simulink library "HANcoder_STM32_Target"  (R2016b)
settings: Solver=ode45  StartTime=0.0  StopTime=10.0  RelTol=1e-3  EnableMultiTasking=on
libraries: simulink x3
(part 4 of 7)

== system HANcoder_STM32_Target/STM32-P405/Digital Outputs ==
  Digital Output : Subsystem  Tag=HANcoder_TARGET_STM32_P405  mask(Digital Output){pinID=Port C pin 12 (LED), config=Push pull, tsamp=-1}
      mask prompts: pinID "Output pin"; config "Configuration"; tsamp "Sample time"
      mask help:
      | Function
      | ========
      | Controls the state of a digital output pin.
      |
      | Parameters
      | ==========
      | Output pin:
      |   Selects the digital output to control
      | Configuration:
      |   Open drain (output float when digital high) or push-pull (output connected
      |   to Vcc when digital high).
      |
      | Inport
      | ==========
      | State of the pin. 0 means logical low and 1 logical high
      mask init:
      | pinIDInfoStr = sfcn_digital_out_mcb(3, pinID, config);
      settings: CopyFcn=sfcn_digital_out_chk();  MoveFcn=drawLogos
      mask Help: web('sfcn_digital_out.html');
      mask TypeOptions pinID: Port A pin 1 | Port A pin 8 | Port B pin 0 | Port B pin 1 | Port B pin 2 | Port B pin 5 | Port B pin 8 | Port B pin 9 | Port B pin 10 | Port B pin 11 | Port B pin 12 | Port B pin 13 | Port B pin 14 | Port B pin 15 | Port C pin 0 | Port C pin 1 | Port C pin 2 | Port C pin 3 | Port C pin 4 | Port C pin 5 | Port C pin 6 | Port C pin 7 | Port C pin 8 | Port C pin 9 | Port C pin 10 | Port C pin 11 | Port C pin 12 (LED) | Port C pin 13 | Port D pin 2
      mask Callback pinID: sfcn_digital_out_chk();
      mask TypeOptions config: Open drain | Push pull
      mask Display: fprintf('Digital Output\n%s', pinIDInfoStr);patch([135 141 141],[8 14 2],[1 0 0]);patch([143 143 149],[14 2 8],[0 0 0.35]);

== system HANcoder_STM32_Target/STM32-P405/Error Handling ==
  Clear errors : Subsystem  Tag=HANcoder_TARGET_STM32_P405  mask(Clear errors){eepromString=Active}
      mask prompts: eepromString "Active or Stored error"
      mask help:
      | [Function]
      | Clears the active(RAM) or stored(EEPROM) errors.
      |
      | [Triggerport]
      | Connect the port to a trigger source to execute the block only when necessary.
      mask init:
      | sfcn_controller_error_clearerrors_mcb(eepromString)
      settings: MoveFcn=drawLogos
      mask Help: web('sfcn_controller_error_clearerrors.html');
      mask TypeOptions eepromString: Active | Stored
      mask Display: fprintf('Clear %s Errors', eepromString);patch([80 86 86],[8 14 2],[1 0 0]);patch([88 88 94],[14 2 8],[0 0 0.35]);
  Delete error : Subsystem  Tag=HANcoder_TARGET_STM32_P405  mask(Delete error){useInPorts=off, errorID=hex2dec('8000'), para=10}
      mask prompts: useInPorts "Use inports"; errorID "Error code"; para "Error parameter"
      mask help:
      | [Function]
      | Delete an error defined by error code and parameter
      | from RAM.
      | Error ID and parameter can be specified in the mask or with inports.
      |
      | [Parameters]
      | Error code
      | Error parameter
      |
      | [Inputs]
      | 1 - Error code [uint16]
      | 2 - Error parameter [uint8]
      |
      | [Triggerport]
      | Connect the port to a trigger source to execute the block only when necessary.
      mask init:
      | sfcn_controller_error_deleteerror_mcb(useInPorts, errorID, para)
      settings: MoveFcn=drawLogos
      mask Help: web('sfcn_controller_error_deleteerror.html');
      mask Display: fprintf('Delete error');patch([80 86 86],[8 14 2],[1 0 0]);patch([88 88 94],[14 2 8],[0 0 0.35]);
  Read active error : Subsystem  Tag=HANcoder_TARGET_STM32_P405  mask(Read active error){tsamp=-1}
      mask prompts: tsamp "Sample time"
      mask help:
      | Function
      | ==========
      | Read an active error from RAM.
      |
      | Inport
      | ==========
      | Input is the number of the error in the error list, which can be 1..64. UINT8
      |
      | Outports
      | ==========
      | 1: UINT8 - total amount of errors.
      | 2: UINT16 - error code.
      | 3: UINT8  - error parameter.
      | 4: UINT8  - occurrence count.
      | 5: UINT32 - last occurrence time since startup [milliseconds].
      |
      | Note that the requested error was set and read only if occurrence count > 0.
      mask init:
      | sfcn_controller_error_readerror_mcb(0)
      settings: MoveFcn=drawLogos
      mask Help: web('sfcn_controller_error_readerror.html');
      mask Display: fprintf('Read active error');patch([80 86 86],[8 14 2],[1 0 0]);patch([88 88 94],[14 2 8],[0 0 0.35]);
  Read stored error : Subsystem  Tag=HANcoder_TARGET_STM32_P405  mask(Read stored error){tsamp=-1}
      mask prompts: tsamp "Sample time"
      mask help:
      | Function
      | ==========
      | Read a stored error from EEPROM.
      |
      | Inport
      | ==========
      | Input is the number of the error in the error list, which can be 1..64. UINT8
      |
      | Outports
      | ==========
      | 1: UINT8 - total amount of errors.
      | 2: UINT16 - error code.
      | 3: UINT8  - error parameter.
      | 4: UINT8  - occurrence count.
      | 5: UINT32 - last occurrence time since startup [milliseconds].
      |
      | Note that the requested error was set and read only if occurrence count > 0.
      mask init:
      | sfcn_controller_error_readerror_mcb(1)
      settings: MoveFcn=drawLogos
      mask Help: web('sfcn_controller_error_readerror.html');
      mask Display: fprintf('Read stored error');patch([80 86 86],[8 14 2],[1 0 0]);patch([88 88 94],[14 2 8],[0 0 0.35]);
  Search active error : Subsystem  Tag=HANcoder_TARGET_STM32_P405  mask(Search active error){tsamp=-1}
      mask prompts: tsamp "Sample time"
      mask help:
      | Function
      | ==========
      | Searches for the erorr with the specified error Code and Param in RAM.
      |
      | Inport
      | ==========
      | 1: UINT16 - Error Code
      | 2: UINT8   - Error Parameter
      |
      | Outports
      | ==========
      | 1: UINT8   - occurrence count.
      | 2: UINT32 - last occurrence time since startup [milliseconds]
      |
      | Note that when occurrence count equals zero, the error is not found.
      mask init:
      | sfcn_controller_error_searcherror_mcb(0)
      settings: MoveFcn=drawLogos
      mask Help: web('sfcn_controller_error_searcherror.html');
      mask Display: fprintf('Search active error');patch([80 86 86],[8 14 2],[1 0 0]);patch([88 88 94],[14 2 8],[0 0 0.35]);
  Search stored error : Subsystem  Tag=HANcoder_TARGET_STM32_P405  mask(Search stored error){tsamp=-1}
      mask prompts: tsamp "Sample time"
      mask help:
      | Function
      | ==========
      | Searches for the erorr with the specified error Code and Param in EEPROM.
      |
      | Inport
      | ==========
      | 1: UINT16 - Error Code
      | 2: UINT8   - Error Parameter
      |
      | Outports
      | ==========
      | 1: UINT8   - occurrence count.
      | 2: UINT32 - last occurrence time since startup [milliseconds]
      |
      | Note that when occurrence count equals zero, the error is not found.
      mask init:
      | sfcn_controller_error_searcherror_mcb(1)
      settings: MoveFcn=drawLogos
      mask Help: web('sfcn_controller_error_searcherror.html');
      mask Display: fprintf('Search stored error');patch([80 86 86],[8 14 2],[1 0 0]);patch([88 88 94],[14 2 8],[0 0 0.35]);
  "Store error " : Subsystem  Tag=HANcoder_TARGET_STM32_P405  mask(Store error){useInPorts=off, errorCode=hex2dec('8000'), parameter=10}
      mask prompts: useInPorts "Use inports"; errorCode "Error code"
      mask help:
      | [Function]
      | Store an error to RAM (and EEPROM if new) of the controller.
      | Error ID and parameter can be specified in the mask or with inports.
      |
      | [Parameters]
      | Error code
      | Error parameter
      |
      | [Inputs]
      | 1 - Error code [uint16]
      | 2 - Error parameter [uint8]
      |
      | [Triggerport]
      | Connect the port to a trigger source to execute the block only when necessary.
      mask init:
      | sfcn_controller_error_storeerror_in_mcb(useInPorts, errorCode, parameter, 1)
      settings: MoveFcn=drawLogos
      mask Help: web('sfcn_controller_error_storeerror.html');
      mask Display: fprintf('Store error');patch([80 86 86],[8 14 2],[1 0 0]);patch([88 88 94],[14 2 8],[0 0 0.35]);
  Total Errors : Subsystem  Tag=HANcoder_TARGET_STM32_P405  mask(Total active or stored errors){eepromString=Active, tsamp=-1}
      mask prompts: eepromString "Active or Stored error"; tsamp "Sample time"
      mask help:
      | [Function]
      | Returns the total amount of active or stored errors
      |
      | [Parameters]
      | Active or Stored error [-]
      | sampleTime: [s]
      |
      | [Outputs]
      | Port 1 :Total number of errors [uint8]
      | Port 2 :Highest occuring severity [uint8]
      mask init:
      | sfcn_controller_error_totalerrors_mcb(eepromString, tsamp);
      settings: MoveFcn=drawLogos
      mask Help: web('sfcn_controller_error_totalerrors.html');
      mask TypeOptions eepromString: Active | Stored
      mask Display: fprintf('Total %s Errors', eepromString);patch([80 86 86],[8 14 2],[1 0 0]);patch([88 88 94],[14 2 8],[0 0 0.35]);

== system HANcoder_STM32_Target/STM32-P405/File Logger ==
  File Logger Close : Subsystem  Tag=HANcoder_TARGET_STM32_P405  mask(File Logger Close){}
      mask help:
      | Function
      | ========
      | With the File Logger module active, the data values of the configured signals
      | are sampled at a fixed time interval and written to the log-file on the SD-card.
      |
      | The log-file needs to be explicitly closed at the end of a logging session for the
      | log-file to actually appear on the SD-card.
      |
      | Ideally, this block is called during software shutdown for example when the ignition
      | signal goes low in automotive applications. An external trigger can also be used such
      | as a button press event or CAN message reception.
      |
      | Triggerport
      | ===========
      | Connect the port to a trigger source to execute the block only when necessary.
      mask init:
      | sfcn_filelogger_close_mcb();
      settings: MoveFcn=drawLogos
      mask Help: web('sfcn_filelogger_close.html')
      mask Display: fprintf('File Logger Close');patch([80 86 86],[8 14 2],[1 0 0]);patch([88 88 94],[14 2 8],[0 0 0.35]);
  File Logger Init : Subsystem  Tag=HANcoder_TARGET_STM32_P405  mask(File Logger Init){filename='mylog.txt', autoincrement=on, firstline='time;signal1;signal2;signal3', interval=100, maxsignals=3, dotseparator=off, autostart=on}
      mask prompts: autoincrement "Add auto-incrementing number to filename"; firstline "First line in log-file"; interval "Logging interval (ms)"; maxsignals "Maximum signals to log"; dotseparator "Use dot-character as decimal separator (comma otherwise)"; autostart "Automatically start logging"
      mask help:
      | Function
      | ==========
      | Initializes the File Logger module.
      |
      | Parameters per channel
      | ======================
      | - Specify filename for the log-file
      | - Select if a 3-digit auto-incrementing number should be added to the log-file
      | - Specify the first line in the log-file
      | - Specify the logging interval in milliseconds
      | - Specify the maximum number of signals to log
      | - Select if a comma or dot should be used a the decimal point in numbers
      | - Select if logging should automatically start after initialization. If not then
      |   a trigger input will appear that can be used to trigger the logging start.
      mask init:
      | sfcn_filelogger_init_mcb(filename, firstline, interval, maxsignals, dotseparator, autoincrement, autostart);
      settings: MoveFcn=drawLogos
      mask Help: web('sfcn_filelogger_init.html')
      mask Display: fprintf('File Logger Init');patch([95 101 101],[8 14 2],[1 0 0]);patch([103 103 109],[14 2 8],[0 0 0.35]);
  File Logger Signal : Subsystem  Tag=HANcoder_TARGET_STM32_P405  mask(File Logger Signal){signalIdx=0, dataType=uint8}
      mask prompts: signalIdx "Signal Index"; dataType "Signal Data Type"
      mask help:
      | Function
      | ==========
      | Configures the signal to be logged by the File Logger module.
      |
      | Parameters per channel
      | ======================
      | - Specify the zero based index of the signal for the File Logger module. In the
      |   File Logger Init block the maximum number of signals was configured
      |   (max_signals). Valid values for this paramter are 0..(max_signals-1).
      | - Select the data type of the signal.
      mask init:
      | sfcn_filelogger_signal_mcb(signalIdx, dataType);
      settings: MoveFcn=drawLogos
      mask Help: web('sfcn_filelogger_signal.html')
      mask TypeOptions dataType: double | single | int8 | uint8 | int16 | uint16 | int32 | uint32
      mask Display: fprintf('File Logger Signal\n(Index %d)', signalIdx);patch([95 101 101],[8 14 2],[1 0 0]);patch([103 103 109],[14 2 8],[0 0 0.35]);

== system HANcoder_STM32_Target/STM32-P405/Memory ==
  EEPROM : Subsystem
      settings: MoveFcn=drawLogos
      mask Display: fprintf('EEPROM');patch([85 91 91],[8 14 2],[1 0 0]);patch([93 93 99],[14 2 8],[0 0 0.35]);

== system HANcoder_STM32_Target/STM32-P405/PWM Outputs ==
  PWM Duty Cycle : Subsystem  Tag=HANcoder_TARGET_STM32_P405  mask(Pulse Width Modulation Set Duty Cycle){pinID=Port A pin 9, tsamp=-1}
      mask prompts: pinID "Output pin"; tsamp "Sample time"
      mask help:
      | Function
      | ========
      | A 'PWM Duty Cycle' block allows the duty cycle of the generated PWM signal to
      | changed.
      | Note that this only works properly if a 'PWM Init' block is also present
      | for initializing the related PWM module.
      |
      | Parameters
      | ==========
      | PWM pin:
      |   Selects the PWM pin for which the duty cycle should be updated.
      |
      | Inport
      | ==========
      | uint16 10-bit unsigned value (0..1023) to represent the duty cycle (0..100%) for
      | each enabled channel.
      mask init:
      | pinIDInfoStr = sfcn_pwmout_setduty_mcb(3, pinID);
      settings: MoveFcn=drawLogos
      mask Help: web('sfcn_pwmout_setduty.html');
      mask TypeOptions pinID: Port A pin 8 | Port A pin 9 | Port A pin 10 | Port A pin 1 | Port C pin 6 | Port C pin 7 | Port C pin 8 | Port C pin 9 | Port B pin 6 | Port B pin 7 | Port B pin 8 | Port B pin 9
      mask Display: fprintf('PWM Set Duty Cycle\n%s', pinIDInfoStr);patch([135 141 141],[8 14 2],[1 0 0]);patch([143 143 149],[14 2 8],[0 0 0.35]);
  PWM Init : Subsystem  Tag=HANcoder_TARGET_STM32_P405  mask(Pulse Width Modulation Initialization){moduleID=TIM1: PA8 & PA9 & PA10 & n/a + N-channels PB13 & PB0 & PB1), frequency=1000, alignment=Edge aligned, enableIRQoutput=off, ch1On=off, ch1Pol=Active high, ch1Inv=off, ch2On=off, ch2Pol=Active high, ch2Inv=off, ch3On=off, ch3Pol=Active high, ch3Inv=off, ch4On=off, ch4Pol=Active high, ch4Inv=off}
      mask prompts: moduleID "PWM module"; frequency "Signal frequency [Hz]"; alignment "Signal alignment"; enableIRQoutput "Enable IRQ output"; ch1On "Generate PWM signal on channel 1"; ch1Pol "Select signal polarity"; ch1Inv "Enable inverted signal on additional output pin"; ch2On "Generate PWM signal on channel 2"; ch2Pol "Select signal polarity"; ch2Inv "Enable inverted signal on additional output pin"; ch3On "Generate PWM signal on channel 3"; ch3Pol "Select signal polarity"; ch3Inv "Enable inverted signal on additional output pin"; ch4On "Generate PWM signal on channel 4"; ch4Pol "Select signal polarity"; ch4Inv "Enable inverted signal on additional output pin"
      mask help:
      | Function
      | ========
      | A 'PWM Init' block configures one of the STM32 timer modules for PWM
      | functionality, allowing a PWM signal to be generated on up to 4 timer
      | channels and their associated output pins.
      |
      | Parameters
      | ==========
      | General - PWM module:
      |   Select the PWM module to use. The name in the combo box contains
      |   information about which pins on the target belong to this timer module.
      |   Also the first pin corresponds with the first channel and so on:
      |   TIMx: Ch1 & Ch2 & Ch3...
      |
      | General - Signal frequency:
      |   Determines the signal frequency in Hz. If you click 'Apply' after entering
      |   the desired frequency it will automatically be adjusted to the closest
      |   supported value.
      |
      | General - Signal Aligment:
      |   Determines the aligment of the signal. It can either be edge aligned or
      |   center aligned.
      |
      | General - Enable IRQ output
      |   Controls whether or not the IRQ output is available.
      |
      | Channel x - Generate PWM signal on channel x:
      |   Enable to configure the channel for PWM functionality so that the PWM signal
      |   is outputted on the channel's associated microcontroller pin.
      |
      | Channel x - Signal polarity:
      |   Selects the polarity of the signal.
      |
      | Channel x - Enable inverted signal on additional output pin:
      |   When enabled, a second PWM signal will be generated on an additional
      |   microcontroller pin where the signal is an exact inversion of the first signal.
      mask init:
      | moduleIDInfoStr = sfcn_pwmout_init_mcb(3, moduleID, frequency, alignment, enableIRQoutput, ch1On, ch2On, ch3On, ch4On, ch1Pol, ch2Pol, ch3Pol, ch4Pol, ch1Inv, ch2Inv, ch3Inv, ch4Inv);
      settings: CopyFcn=sfcn_pwmout_init_chk();  MoveFcn=drawLogos
      mask Help: web('sfcn_pwmout_init.html');
      mask TypeOptions moduleID: TIM1: PA8 & PA9 & PA10 & n/a + N-channels PB13 & PB0 & PB1) | TIM2:n/a & PA1 & n/a & n/a | TIM3: PC6 & PC7 & PC8 & PC9 | TIM4: PB6 & PB7 & PC8 & PB9
      mask Callback moduleID: sfcn_pwmout_init_chk();
      mask TypeOptions alignment: Edge aligned | Center aligned
      mask TypeOptions ch1Pol: Active high | Active low
      mask TypeOptions ch2Pol: Active high | Active low
      mask TypeOptions ch3Pol: Active high | Active low
      mask TypeOptions ch4Pol: Active high | Active low
      mask Display: fprintf('PWM Init\n%s', moduleIDInfoStr);patch([185 191 191],[8 14 2],[1 0 0]);patch([193 193 199],[14 2 8],[0 0 0.35]);

== system HANcoder_STM32_Target/STM32-P405/SPI ==
  SPI master init : Subsystem  Tag=HANcoder_TARGET_STM32_P405  mask(SPI master init){channel=SPI1: UEXT 9 & 7 & 8 (PA5 & PA6 & PA7), speed=5250 kHz, polarity=Idle low, phase=Sample bit on 1st clock edge}
      mask prompts: speed "Communication speed"
      mask help:
      | Function
      | ==========
      | Initialized a SPI master channel.
      |
      | Parameters per channel
      | ======================
      | - Select channel
      | - Select communication speed
      | - Select clock signal polarity
      | - Select clock phase to sample a bit
      mask init:
      | spiChannelInfoStr = sfcn_spi_master_init_mcb(3, channel, speed, polarity, phase);
      settings: CopyFcn=sfcn_spi_master_init_chk();  MoveFcn=drawLogos
      mask Help: web('sfcn_spi_master_init.html')
      mask TypeOptions channel: SPI1: UEXT 9 & 7 & 8 (PA5 & PA6 & PA7) | SPI2: PB13 & PB14 & PB15
      mask Callback channel: sfcn_spi_master_init_chk();
      mask TypeOptions speed: 21000 kHz | 10500 kHz | 5250 kHz | 2625 kHz | 1312.5 kHz | 656.25 kHz | 328.125 kHz | 164.0625 kHz
      mask TypeOptions polarity: Idle low | Idle high
      mask TypeOptions phase: Sample bit on 1st clock edge | Sample bit on 2nd clock edge
      mask Display: fprintf('SPI master init\n%s', spiChannelInfoStr);patch([211 217 217],[8 14 2],[1 0 0]);patch([219 219 225],[14 2 8],[0 0 0.35]);
  SPI master transfer : Subsystem  Tag=HANcoder_TARGET_STM32_P405  mask(SPI master transfer){channel=SPI1: UEXT 9 & 7 & 8 (PA5 & PA6 & PA7), useSS=off, SSpin=Port A pin 1, SSenable=on, SSdisable=on, delayCycles=0, tsamp=-1}
      mask prompts: useSS "Use slave select output"; SSpin "Slave select output pin"; SSenable "Enable slave select before transfer"; SSdisable "Disable slave select after transfer"; delayCycles "Delay cycles between slave select enable and transfer"; tsamp "Sample time"
      mask help:
      | Function
      | ==========
      | Performs a byte transfer via SPI.
      |
      | Parameters per channel
      | ======================
      | - Select channel
      | - Select if a Slave Select output should be controlled
      |   * Select the Slave Select digital output pin
      |   * Select if the Slave Select should be made logic low before the transfer
      |   * Select if the Slave Select should be made logic high after the transfer
      |   * Enter the number of CPU cycles to delay between Slave Select enable and the transfer
      |
      | Inputs
      | ======
      | The byte value to send to the slave.
      |
      | Outputs
      | =======
      | The byte value received from the slave.
      mask init:
      | spiChannelInfoStr = sfcn_spi_master_transfer_mcb(3, channel, useSS, SSpin, SSenable, SSdisable, delayCycles);
      settings: MoveFcn=drawLogos
      mask Help: web('sfcn_spi_master_transfer.html')
      mask TypeOptions channel: SPI1: UEXT 9 & 7 & 8 (PA5 & PA6 & PA7) | SPI2: PB13 & PB14 & PB15
      mask TypeOptions SSpin: Port A pin 1 | Port A pin 8 | Port B pin 0 | Port B pin 1 | Port B pin 2 | Port B pin 5 | Port B pin 8 | Port B pin 9 | Port B pin 10 | Port B pin 11 | Port B pin 12 | Port B pin 13 | Port B pin 14 | Port B pin 15 | Port C pin 0 | Port C pin 1 | Port C pin 2 | Port C pin 3 | Port C pin 4 | Port C pin 5 | Port C pin 6 | Port C pin 7 | Port C pin 8 | Port C pin 9 | Port C pin 10 | Port C pin 11 | Port C pin 12 (LED) | Port C pin 13 | Port D pin 2
      mask Display: fprintf('SPI master transfer\n%s', spiChannelInfoStr);patch([210 216 216],[8 14 2],[1 0 0]);patch([218 218 224],[14 2 8],[0 0 0.35]);

== system HANcoder_STM32_Target/STM32-P405/System Config ==
  Base Sample Time config : Subsystem  Tag=HANcoder_TARGET_STM32_P405  Description=HANcoder Target STM32-P405 blockset version 0.5  mask(Base Sample Time config){baseSampleTime=10, extraStack=100}
      mask prompts: baseSampleTime "Define the base sample time [ms]"; extraStack "Additional task stack (bytes):"
      mask help:
      | Function
      | ==========
      | Sets the Base Sample Time in the model, and automatically sets the sample
      | time in the solver step time menu when the model is simulated or build.
      |
      | Parameters
      | ==========
      | Base Sample Time [milliseconds]
      | Default:    10[ms]
      | Min:        0.1[ms]
      |
      | Note: This is the only block where sample time is set in miliseconds,
      | all other blocks work with sample time in seconds
      |
      | It is possible to reserve extra stack space for the OS task that executes
      | the model on the embedded target (AppCtrlTask).
      mask init:
      | sfcn_base_sample_time_mcb(baseSampleTime*1000, extraStack, 3);
      | HANcoderStruct = get_param(gcb,'UserData');
      | BlocksetVersion = HANcoderStruct.BlocksetVersion;
      settings: MoveFcn=drawLogos
      mask Help: web('sfcn_base_sample_time.html')
      mask Display: fprintf('Blockset version %s\nBase Sample Time:\n %gms',BlocksetVersion,baseSampleTime);patch([91 97 97],[8 14 2],[1 0 0]);patch([99 99 105],[14 2 8],[0 0 0.35]);
  Build settings : Subsystem  Tag=HANcoder_TARGET_STM32_P405  mask(Build Settings){AutoASAP2add=on, AutoFlash=USB}
      mask prompts: AutoASAP2add "Add signals and parameters automatically"; AutoFlash "Automatic flash after build"
      mask help:
      | Function
      | ==========
      | Auto Add:
      | Here you can turn the automatic adding of Signals and Parameters on or off. If the option is on all the parameters and signals which are not defined in the workspace will be added. You will be prompted for the value.
      |
      | Auto Flash:
      | This option will automatically start MicroBoot with the selected interface.
      settings: MoveFcn=drawLogos
      mask Help: web('build_settings.html')
      mask TypeOptions AutoASAP2add: on | off
      mask TypeOptions AutoFlash: off | USB | CAN
      mask DialogControl Control3 Prompt: With this option the undefined parameters and signals will automatically be added to the workspace for use with HANtune. You will be prompted for the parameter values.
      mask DialogControl Control2 Prompt: With this option you can choose to automatically start MicroBoot after the build is complete. MicroBoot will start flashing using the selected interface.
      mask Display: fprintf('Build settings\nAuto Add: %s\nAuto Flash: %s',AutoASAP2add, AutoFlash);patch([114 120 120],[8 14 2],[1 0 0]);patch([122 122 128],[14 2 8],[0 0 0.35]);
  CAN config : Subsystem  Tag=HANcoder_TARGET_STM32_P405  mask(CAN config){txBufSize=64, evBufSize=64, canBus1=on, baudRate1=500, rxMask1=hex2dec('00000000'), rxCode1=hex2dec('00000000'), rxMode1=Receive only 11-bit message identifiers, canBus2=off, baudRate2=500, rxMask2=hex2dec('00000000'), rxCode2=hex2dec('00000000'), rxMode2=Receive only 11-bit message identifiers}
      mask prompts: txBufSize "Transmit buffer size CAN bus (max 512)"; evBufSize "Event buffer size CAN bus"; canBus1 "Use CAN bus 1"; baudRate1 "Baudrate CAN bus 1 (kbit/s)"; rxMask1 "Reception filter Mask CAN bus 1"; rxCode1 "Reception filter Code CAN bus 1"; rxMode1 "Reception filter Mode CAN bus 1"; canBus2 "Use CAN bus 2"; baudRate2 "Baudrate CAN bus 2 (kbit/s)"; rxMask2 "Reception filter Mask CAN bus 2"; rxCode2 "Reception filter Code CAN bus 2"; rxMode2 "Reception filter Mode CAN bus 2"
      mask help:
      | Function
      | ==========
      | Configures the settings for the STM32's CAN busses.
      |
      | Parameters per channel
      | ======================
      | - Activate channel
      | - Select baud rate (default 500[kbit/s])
      | - Select reception acceptance filter Code
      | - Select reception acceptance filter Mask
      | - Select reception acceptance filter Mode
      mask init:
      | sfcn_can_config_mcb(txBufSize, evBufSize, canBus1, baudRate1, rxMask1, rxCode1, rxMode1, canBus2, baudRate2, rxMask2, rxCode2, rxMode2);
      settings: MoveFcn=drawLogos
      mask Help: web('sfcn_can_config.html')
      mask TypeOptions baudRate1: 125 | 250 | 500 | 1000
      mask TypeOptions rxMode1: Receive only 11-bit message identifiers | Receive only 29-bit message identifiers | Received both 11- and 29-bit message identifiers
      mask TypeOptions baudRate2: 125 | 250 | 500 | 1000
      mask TypeOptions rxMode2: Receive only 11-bit message identifiers | Receive only 29-bit message identifiers | Received both 11- and 29-bit message identifiers
      mask Display: fprintf('CAN1 : %x\nCAN2 : %x',canBus1, canBus2);patch([58 64 64],[8 14 2],[1 0 0]);patch([66 66 72],[14 2 8],[0 0 0.35]);
  Custom ID config : Subsystem  Tag=HANcoder_TARGET_STM32_P405  mask(Custom ID config){softID=softwareID, softNUM=1}
      mask prompts: softID "Software ID Name"; softNUM "Software Version Number"
      mask help:
      | Function:
      | =========
      | This block can be used to override the generated software ID as the current software version which is used for identification purposes.
      | It can also be used to add a version number behind the software ID.
      |
      | Details:
      | ========
      | If only a software version number is filled in, a software ID will be generated and the version number will be placed behind it.
      | Atleast one pf the fields has to be filled in.
      |
      | Parameters:
      | ===========
      | Software ID name:
      | Fill in the desired custom ID. Must fit in a UINT8
      | Software Version Number:
      | Fill in the desired version number. Must fit in a UINT8
      mask init:
      | sfcn_custom_version_config_mcb(softID, softNUM)
      settings: MoveFcn=drawLogos
      mask Help: web('sfcn_custom_ID_config.html')
      mask Display: fprintf('Custom software ID:\n "%s"\n Software version:\n "%s"', char(softID), char(softNUM));patch([112 118 118],[8 14 2],[1 0 0]);patch([120 120 126],[14 2 8],[0 0 0.35]);
  XCP on CAN config : Subsystem  Tag=HANcoder_TARGET_STM32_P405  mask(XCP on CAN config){canBus=CAN 1, croID=hex2dec('665'), dtoID=hex2dec('666')}
      mask prompts: canBus "CAN channel"; croID "CRO identifier"; dtoID "DTO identifier"
      mask help:
      | Function
      | ==========
      | Implements XCP communication into your application using the CAN network.
      |
      | Parameter
      | ==========
      | Specify the CAN channel to be used for XCP.
      | Specify the CAN CRO message identifier for XCP (master->slave).
      | Specify the CAN DTO message identifier for XCP (slave->master).
      |
      | Notes
      | ==========
      | Baudrates can be modified in the CAN config block.
      mask init:
      | sfcn_can_xcp_config_mcb(canBus, croID, dtoID)
      settings: MoveFcn=drawLogos
      mask Help: web('sfcn_can_xcp_config.html')
      mask TypeOptions canBus: CAN 1 | CAN 2
      mask Display: fprintf('XCP over CAN: %x',canBus);patch([69 75 75],[8 14 2],[1 0 0]);patch([77 77 83],[14 2 8],[0 0 0.35]);
  XCP on USB config : Subsystem  Tag=HANcoder_TARGET_STM32_P405  mask(XCP on USB config){}
      mask help:
      | Function
      | ==========
      | Implements XCP communication into your application using the USB Virtual COM-port.
      mask init:
      | sfcn_usb_xcp_config_mcb()
      settings: MoveFcn=drawLogos
      mask Help: web('sfcn_usb_xcp_config.html')
      mask Display: fprintf('XCP over USB');patch([69 75 75],[8 14 2],[1 0 0]);patch([77 77 83],[14 2 8],[0 0 0.35]);

== system HANcoder_STM32_Target/STM32-P405/System Management ==
  Enter Critical Section : Subsystem  Tag=HANcoder_TARGET_STM32_P405  mask(Enter a critical section){tsamp=-1}
      mask prompts: tsamp "Sample time"
      mask help:
      | Function
      | ==========
      | Enters a critical section that can not be interrupted. This block must
      | always be used in a pair together with "Exit Critical Section". Click the
      | Help-button for a detailed example on how to use this block.
      mask init:
      | sfcn_critical_enter_mcb();
      settings: MoveFcn=drawLogos
      mask Help: web('sfcn_critical_section.html');
      mask Display: fprintf('Enter Critical Section');patch([95 101 101],[8 14 2],[1 0 0]);patch([103 103 109],[14 2 8],[0 0 0.35]);
  Exit Critical Section : Subsystem  Tag=HANcoder_TARGET_STM32_P405  mask(Exit a critical section){tsamp=-1}
      mask prompts: tsamp "Sample time"
      mask help:
      | Function
      | ==========
      | Exits a critical section. This block must always be used in a pair together
      | with "Enter Critical Section". Click the Help-button for a detailed example
      | on how to use this block.
      mask init:
      | sfcn_critical_exit_mcb();
      settings: MoveFcn=drawLogos
      mask Help: web('sfcn_critical_section.html');
      mask Display: fprintf('Exit Critical Section');patch([95 101 101],[8 14 2],[1 0 0]);patch([103 103 109],[14 2 8],[0 0 0.35]);
  Get CPU load : Subsystem  Tag=HANcoder_TARGET_STM32_P405  mask(Get CPU load){mode=Current CPU load, tsamp=-1}
      mask prompts: tsamp "Sample time"
      mask help:
      | Function
      | ==========
      | Get the CPU load of the system.
      |
      | Parameters
      | ==========
      | Mode specifies if the current CPU load should be read or the maximum CPU
      | load since reset.
      |
      | Outport
      | ==========
      | CPU load as a percentage.
      mask init:
      | if mode==1
      |   modeStr = 'current';
      | else
      |   modeStr = 'maximum';
      | end
      | sfcn_controller_cpu_getload_mcb(mode);
      settings: MoveFcn=drawLogos
      mask Help: web('sfcn_controller_cpu_getload.html');
      mask TypeOptions mode: Current CPU load | Maximum CPU load
      mask Display: fprintf('Get %s\nCPU load', modeStr);patch([95 101 101],[8 14 2],[1 0 0]);patch([103 103 109],[14 2 8],[0 0 0.35]);
  Get free Heap : Subsystem  Tag=HANcoder_TARGET_STM32_P405  mask(Get free Heap){tsamp=-1}
      mask prompts: tsamp "Sample time"
      mask help:
      | Function
      | ==========
      | Obtains the number of bytes that are still available on the heap.
      |
      | Outport
      | ==========
      | Number of bytes that are still available on the heap.
      mask init:
      | sfcn_controller_getheap_mcb();
      settings: MoveFcn=drawLogos
      mask Help: web('sfcn_controller_getheap.html');
      mask Display: fprintf('Get free Heap');patch([95 101 101],[8 14 2],[1 0 0]);patch([103 103 109],[14 2 8],[0 0 0.35]);
  Get free Stack : Subsystem  Tag=HANcoder_TARGET_STM32_P405  mask(Get free Stacl){taskIdx=Application Control Task, tsamp=-1}
      mask prompts: taskIdx "Task name"; tsamp "Sample time"
      mask help:
      | Function
      | ========
      | Obtains the number of bytes that are still available on the stack of a particular task.
      |
      | Parameter
      | =========
      | Name of the task for which the free stack space should be read.
      |
      | Outport
      | =======
      | Number of bytes that are still available on the task's stack.
      mask init:
      | sfcn_controller_getstack_mcb(taskIdx);
      settings: MoveFcn=drawLogos
      mask Help: web('sfcn_controller_getstack.html');
      mask TypeOptions taskIdx: Idle Task | Timer Task | Can Event Task | Can Transmit Task | Application Control Task | Measurement and Calibration Network Task
      mask Display: fprintf('Get free Stack');patch([95 101 101],[8 14 2],[1 0 0]);patch([103 103 109],[14 2 8],[0 0 0.35]);
  Reset ECU : Subsystem  Tag=HANcoder_TARGET_STM32_P405  mask(Reset ECU){}
      mask help:
      | Function
      | ==========
      | Triggering this block causes the ECU to reset.
      mask init:
      | sfcn_controller_reset_mcb()
      settings: MoveFcn=drawLogos
      mask Help: web('sfcn_controller_reset.html');
      mask Display: fprintf('Reset ECU');patch([60 66 66],[8 14 2],[1 0 0]);patch([68 68 74],[14 2 8],[0 0 0.35]);

== system HANcoder_STM32_Target/STM32-P405/Timer Inputs ==
  Quadrature Encoder Get : Subsystem  Tag=HANcoder_TARGET_STM32_P405  mask(Quadrature Encoder Inputs){moduleID=TIM3: PORTC PIN6 & PORTC PIN7 - 5V Tolerant, config=Floating, counterReset=off, tsamp=-1}
      mask prompts: moduleID "Quad encoder module"; config "Configuration"; counterReset "Show counter reset input"; tsamp "Sample time"
      mask help:
      | Function
      | ========
      | Reads the counter of the quadrature encoder module.
      |
      | Parameters
      | ==========
      | Quadrature encoder module:
      |   Selects the quadrature encoder module. The channel A and B signals of the
      |   encoder should be connected to the 2 input pins that belong to the module.
      |
      | Configuration:
      |   Determines if the input is floating or is connected to an internal
      |   pull-up or pull-down resistor.
      |
      | Show counter reset input:
      |   Configures if the input port for the counter reset should be shown.
      |
      |
      | Outport
      | ==========
      | 32-bit signed counter. The counter starts at zero and counts up or down
      | depending on the direction of the motor.
      mask init:
      | moduleIDInfoStr = sfcn_quad_encoder_get_mcb(3,moduleID, counterReset, config);
      settings: CopyFcn=sfcn_quad_encoder_get_chk();  MoveFcn=drawLogos
      mask Help: web('sfcn_quad_encoder_get.html');
      mask TypeOptions moduleID: TIM1: PORTA PIN8 & PORTA PIN9 - 5V Tolerant | TIM3: PORTC PIN6 & PORTC PIN7 - 5V Tolerant | TIM4: PORTB PIN6 & PORTB PIN7 - 5V Tolerant
      mask Callback moduleID: sfcn_quad_encoder_get_chk();
      mask TypeOptions config: Floating | Pullup | Pulldown
      mask Display: fprintf('Quad Encoder Get\n%s', moduleIDInfoStr);patch([135 141 141],[8 14 2],[1 0 0]);patch([143 143 149],[14 2 8],[0 0 0.35]);
  Timer Input Get : Subsystem  Tag=HANcoder_TARGET_STM32_P405  mask(Timer Input Get){pin=TIM1: Con. PA8 (PORTA PIN8) - 5V Tolerant, zeroHzTimeoutMs=2000, tsamp=-1}
      mask prompts: pin "Timer input pin"; zeroHzTimeoutMs "0 Hz detection time (ms)"; tsamp "Sample time"
      mask help:
      | Function
      | ========
      | Reads the information from a timer input pin.
      |
      | Parameters
      | ==========
      | Timer input pin:
      |   Selects the timer input pin.
      |
      | Zero Hz detection time:
      |   Determines after how many milliseconds since the last edge the 0 Hz
      |   detected output flag should go high.
      |
      | Outport
      | ==========
      | Frequency
      |   The last measured frequency on the pin in Hz.
      |
      | Duty cycle
      |   The last measured duty cycle on the pin as a % with a scaling factor of 100 for
      |   improved resolution. So 5000 = 50% for example.
      |
      | Edge count
      |   The number of edges that were detected on the input pin since startup.
      |
      | Edge timestamp
      |   A 32-bit timestamp value of the last edge. The timestamp is derived from an
      |   internal 32-bit free running counter that runs at 21 Mhz.
      |
      | 0 Hz detected
      |   A boolean flag that will go high if no edges were detected for the time specified
      |   as the zero Hz detection time. Upon the next edge the flag will go low again.
      mask init:
      | timeinPinIdInfoStr = sfcn_timein_get_mcb(3, pin, zeroHzTimeoutMs);
      settings: CopyFcn=sfcn_timein_get_chk();  MoveFcn=drawLogos
      mask Help: web('sfcn_timein_get.html');
      mask TypeOptions pin: TIM1: Con. PA8 (PORTA PIN8) - 5V Tolerant | TIM1: Con. UEXT-3 (PORTA PIN9) - 5V Tolerant | TIM1: Con. UEXT-4 (PORTA PIN10) - 5V Tolerant | TIM2: Con. PA1 (PORTA PIN1) - 5V Tolerant | TIM3: Con. PC6 (PORTC PIN6) - 5V Tolerant | TIM3: Con. PC7 (PORTC PIN7) - 5V Tolerant | TIM3: Con. PC8 (PORTC PIN8) - 5V Tolerant | TIM3: Con. PC9 (PORTC PIN9) - 5V Tolerant | TIM4: Con. UEXT-5 (PORTB PIN6) - 5V Tolerant | TIM4: Con. UEXT-6 (PORTB PIN7) - 5V Tolerant | TIM4: Con. PB8 (PORTB PIN8) - 5V Tolerant | TIM4: Con. PB9 (PORTB PIN9) - 5V Tolerant
      mask Callback pin: sfcn_timein_get_chk();
      mask Display:
      | fprintf('Timer Input Get\n%s', timeinPinIdInfoStr);
      | port_label('output', 1, 'Frequency');
      | port_label('output', 2, 'Duty cycle');
      | port_label('output', 3, 'Edge count');
      | port_label('output', 4, 'Edge state');
      | port_label('output', 5, 'Edge timestamp');
      | port_label('output', 6, 'Counter timestamp');
      | port_label('output', 7, '0 Hz detected');patch([250 256 256],[8 14 2],[1 0 0]);patch([258 258 264],[14 2 8],[0 0 0.35]);
  Timer Input IRQ : Subsystem  Tag=HANcoder_TARGET_STM32_P405  mask(Timer Input IRQ){pin=TIM1: Con. PA8 (PORTA PIN8) - 5V Tolerant}
      mask prompts: pin "Timer input pin"
      mask help:
      | Function
      | ========
      | Enables a function call subsystem to be connected that is executed on interrupt level
      | each time an edge change on the input pin was detected.
      |
      | Parameters
      | ==========
      | Timer input pin:
      |   Selects the timer input pin.
      |
      | Outport
      | =======
      | IRQ
      |   Allows connection of a function call subsystem.
      mask init:
      | timeinPinIdInfoStr = sfcn_timein_irq_mcb(3, pin);
      settings: CopyFcn=sfcn_timein_irq_chk();  MoveFcn=drawLogos
      mask Help: web('sfcn_timein_irq.html');
      mask TypeOptions pin: TIM1: Con. PA8 (PORTA PIN8) - 5V Tolerant | TIM1: Con. UEXT-3 (PORTA PIN9) - 5V Tolerant | TIM1: Con. UEXT-4 (PORTA PIN10) - 5V Tolerant | TIM2: Con. PA1 (PORTA PIN1) - 5V Tolerant | TIM3: Con. PC6 (PORTC PIN6) - 5V Tolerant | TIM3: Con. PC7 (PORTC PIN7) - 5V Tolerant | TIM3: Con. PC8 (PORTC PIN8) - 5V Tolerant | TIM3: Con. PC9 (PORTC PIN9) - 5V Tolerant | TIM4: Con. UEXT-5 (PORTB PIN6) - 5V Tolerant | TIM4: Con. UEXT-6 (PORTB PIN7) - 5V Tolerant | TIM4: Con. PB8 (PORTB PIN8) - 5V Tolerant | TIM4: Con. PB9 (PORTB PIN9) - 5V Tolerant
      mask Callback pin: sfcn_timein_irq_chk();
      mask Display: fprintf('Timer Input IRQ\n%s', timeinPinIdInfoStr);patch([250 256 256],[8 14 2],[1 0 0]);patch([258 258 264],[14 2 8],[0 0 0.35]);

== system HANcoder_STM32_Target/STM32-P405/Timer Outputs ==
  Compare Event IRQ : Subsystem  Tag=HANcoder_TARGET_STM32_P405  mask(Compare Event IRQ){pin=TIM1: Con. PA8 (PORTA PIN8) - 5V Tolerant}
      mask prompts: pin "Timer output pin"
      mask help:
      | Function
      | ========
      | Enables a function call subsystem to be connected that is executed on interrupt
      | level each time an output compare event was triggered.
      |
      | Parameters
      | ==========
      | Timer Output Pin:
      |   Selects the timer channel.
      |
      | Outport
      | =======
      | IRQ
      |   Allows connection of a function call subsystem.
      mask init:
      | timeoutPinIdInfoStr = sfcn_timeout_event_irq_mcb(3, pin);
      settings: CopyFcn=sfcn_timeout_event_irq_chk();  MoveFcn=drawLogos
      mask Help: web('sfcn_timeout_event_irq.html');
      mask TypeOptions pin: TIM1: Con. PA8 (PORTA PIN8) - 5V Tolerant | TIM1: Con. UEXT-3 (PORTA PIN9) - 5V Tolerant | TIM1: Con. UEXT-4 (PORTA PIN10) - 5V Tolerant | TIM2: Con. PA1 (PORTA PIN1) - 5V Tolerant | TIM3: Con. PC6 (PORTC PIN6) - 5V Tolerant | TIM3: Con. PC7 (PORTC PIN7) - 5V Tolerant | TIM3: Con. PC8 (PORTC PIN8) - 5V Tolerant | TIM3: Con. PC9 (PORTC PIN9) - 5V Tolerant | TIM4: Con. UEXT-5 (PORTB PIN6) - 5V Tolerant | TIM4: Con. UEXT-6 (PORTB PIN7) - 5V Tolerant | TIM4: Con. PB8 (PORTB PIN8) - 5V Tolerant | TIM4: Con. PB9 (PORTB PIN9) - 5V Tolerant
      mask Callback pin: sfcn_timeout_event_irq_chk();
      mask Display: fprintf('Compare Event IRQ\n%s', timeoutPinIdInfoStr);patch([135 141 141],[8 14 2],[1 0 0]);patch([143 143 149],[14 2 8],[0 0 0.35]);
  Get Free Running Counter : Subsystem  Tag=HANcoder_TARGET_STM32_P405  mask(Get Free Running Counter){moduleID=TIM1, tsamp=-1}
      mask prompts: moduleID "Timer module"; tsamp "Sample time"
      mask help:
      | Function
      | ========
      | Reads the timer module's internal 16-bit free running counter value.
      |
      | Parameters
      | ==========
      | Timer Module:
      |   Selects the timer module.
      |
      | Outport
      | =======
      | 16-bit free running counter value.
      mask init:
      | moduleIDInfoStr = sfcn_timeout_getrunningcounter_mcb(3, moduleID);
      settings: MoveFcn=drawLogos
      mask Help: web('sfcn_timeout_getrunningcounter.html');
      mask TypeOptions moduleID: TIM1 | TIM2 | TIM3 | TIM4
      mask Display: fprintf('Get Free Running Counter\n%s', moduleIDInfoStr);patch([135 141 141],[8 14 2],[1 0 0]);patch([143 143 149],[14 2 8],[0 0 0.35]);
  Get Last Event Counter : Subsystem  Tag=HANcoder_TARGET_STM32_P405  mask(Get Last Event Counter){pin=TIM1: Con. PA8 (PORTA PIN8) - 5V Tolerant, tsamp=-1}
      mask prompts: pin "Timer output pin"; tsamp "Sample time"
      mask help:
      | Function
      | ========
      | Reads the timer channel's timestamp of the 16-bit free running counter
      | value at which the last output compare event occurred.
      |
      | Parameters
      | ==========
      | Timer Output Pin:
      |   Selects the timer channel.
      |
      | Outport
      | =======
      | 16-bit free running counter timestamp of the last output compare event.
      mask init:
      | timeoutPinIdInfoStr = sfcn_timeout_getlasteventcounter_mcb(3, pin);
      settings: MoveFcn=drawLogos
      mask Help: web('sfcn_timeout_getlasteventcounter.html');
      mask TypeOptions pin: TIM1: Con. PA8 (PORTA PIN8) - 5V Tolerant | TIM1: Con. UEXT-3 (PORTA PIN9) - 5V Tolerant | TIM1: Con. UEXT-4 (PORTA PIN10) - 5V Tolerant | TIM2: Con. PA1 (PORTA PIN1) - 5V Tolerant | TIM3: Con. PC6 (PORTC PIN6) - 5V Tolerant | TIM3: Con. PC7 (PORTC PIN7) - 5V Tolerant | TIM3: Con. PC8 (PORTC PIN8) - 5V Tolerant | TIM3: Con. PC9 (PORTC PIN9) - 5V Tolerant | TIM4: Con. UEXT-5 (PORTB PIN6) - 5V Tolerant | TIM4: Con. UEXT-6 (PORTB PIN7) - 5V Tolerant | TIM4: Con. PB8 (PORTB PIN8) - 5V Tolerant | TIM4: Con. PB9 (PORTB PIN9) - 5V Tolerant
      mask Display: fprintf('Get Last Event Counter\n%s', timeoutPinIdInfoStr);patch([135 141 141],[8 14 2],[1 0 0]);patch([143 143 149],[14 2 8],[0 0 0.35]);
  Output Compare Init : Subsystem  Tag=HANcoder_TARGET_STM32_P405  mask(Output Compare Init){moduleID=TIM1: PA8 & PA9 & PA10 & n/a, frequency=2000000, enableIRQoutput=off}
      mask prompts: moduleID "Timer module"; frequency "Frequency (free running counter) [Hz]"; enableIRQoutput "Enable IRQ output"
      mask help:
      | Function
      | ========
      | Initializes the timer module to allow output compare functionality on the
      | module's channels.
      |
      | Parameters
      | ==========
      | Timer Module:
      |   Selects the timer module.
      |
      | Frequency:
      |   Frequency at which the 16-bit free running counter counts.
      |
      | Enable IRQ output
      |   Controls whether or not the IRQ output is available.
      |
      | Outport
      | =======
      | IRQ
      |   Allows connection of a function call subsystem for the free running
      |   counter overflow event.
      mask init:
      | moduleIDInfoStr = sfcn_timeout_init_mcb(3, moduleID, frequency, enableIRQoutput);
      settings: CopyFcn=sfcn_timeout_init_chk();  MoveFcn=drawLogos
      mask Help: web('sfcn_timeout_init.html');
      mask TypeOptions moduleID: TIM1: PA8 & PA9 & PA10 & n/a | TIM2: n/a & PA1 & n/a & n/a | TIM3: PC6 & PC7 & PC8 & PC9 | TIM4: PB6 & PB7 & PC8 & PB9
      mask Callback moduleID: sfcn_timeout_init_chk();
      mask Display: fprintf('Output Compare Init\n%s', moduleIDInfoStr);patch([135 141 141],[8 14 2],[1 0 0]);patch([143 143 149],[14 2 8],[0 0 0.35]);
  Reset Free Running Counter : Subsystem  Tag=HANcoder_TARGET_STM32_P405  mask(Reset Free Running Counter){moduleID=TIM1}
      mask prompts: moduleID "Timer module"
      mask help:
      | Function
      | ========
      | Resets the value of the timer module's 16-bit free running counter back to
      | 0.
      |
      | Triggerport
      | ===========
      | Connect the port to a trigger source to execute the block only when necessary.
      mask init:
      | moduleIDInfoStr = sfcn_timeout_resetcounter_mcb(3, moduleID);
      settings: MoveFcn=drawLogos
      mask Help: web('sfcn_timeout_resetcounter.html');
      mask TypeOptions moduleID: TIM1 | TIM2 | TIM3 | TIM4
      mask Display: fprintf('Reset Free Running Counter\n%s', moduleIDInfoStr);patch([132 138 138],[8 14 2],[1 0 0]);patch([140 140 146],[14 2 8],[0 0 0.35]);
  Schedule Compare Event : Subsystem  Tag=HANcoder_TARGET_STM32_P405  mask(Schedule Compare Event){pin=TIM1: Con. PA8 (PORTA PIN8) - 5V Tolerant, tsamp=-1}
      mask prompts: pin "Timer output pin"; tsamp "Sample time"
      mask help:
      | Function
      | ========
      | Schedules the next output compare event. The first input determines the
      | value of the timer module's 16-bit free running counter when the event
      | should trigger. The second input determines the action that should
      | be taken on the timer channel's pin.
      |
      | Parameters
      | ==========
      | Timer output pin:
      |   Selects the timer channel's pin.
      |
      | Inport
      | ======
      | Counter
      |   Value of the timer module's 16-bit free running counter at which the
      |   event should trigger.
      |
      | Action
      |   Action to take on the channel's pin when the event triggers:
      |   0: set output pin to logic low.
      |   1: set output pin to logic high.
      |   2: invert logic state of the outpin pin.
      |   3: do nothing to the output pin.
      mask init:
      | timeoutPinIdInfoStr = sfcn_timeout_scheduleevent_mcb(3, pin);
      settings: MoveFcn=drawLogos
      mask Help: web('sfcn_timeout_scheduleevent.html');
      mask TypeOptions pin: TIM1: Con. PA8 (PORTA PIN8) - 5V Tolerant | TIM1: Con. UEXT-3 (PORTA PIN9) - 5V Tolerant | TIM1: Con. UEXT-4 (PORTA PIN10) - 5V Tolerant | TIM2: Con. PA1 (PORTA PIN1) - 5V Tolerant | TIM3: Con. PC6 (PORTC PIN6) - 5V Tolerant | TIM3: Con. PC7 (PORTC PIN7) - 5V Tolerant | TIM3: Con. PC8 (PORTC PIN8) - 5V Tolerant | TIM3: Con. PC9 (PORTC PIN9) - 5V Tolerant | TIM4: Con. UEXT-5 (PORTB PIN6) - 5V Tolerant | TIM4: Con. UEXT-6 (PORTB PIN7) - 5V Tolerant | TIM4: Con. PB8 (PORTB PIN8) - 5V Tolerant | TIM4: Con. PB9 (PORTB PIN9) - 5V Tolerant
      mask Display: fprintf('Schedule Compare Event\n%s', timeoutPinIdInfoStr);patch([135 141 141],[8 14 2],[1 0 0]);patch([143 143 149],[14 2 8],[0 0 0.35]);

== system HANcoder_STM32_Target/STM32-P405/UART ==
  UART init : Subsystem  Tag=HANcoder_TARGET_STM32_P405  mask(UART init){channel=UART1: Con. UEXT-3 & Con. UEXT-4 (PA9 & PA10), baudrate=19200, databits=8, parity=none, stopbits=1, txbufsize=32, rxbufsize=32, useStatusOut=off}
      mask prompts: baudrate "Baudrate (bit/s)"; txbufsize "Transmit buffer size"; rxbufsize "Receive buffer size"; useStatusOut "Use status output"
      mask help:
      | Function
      | ==========
      | Initialized a UART channel.
      |
      | Parameters per channel
      | ======================
      | - Select channel
      | - Select baudrate
      | - Select number of databits
      | - Select parity
      | - Select number of stopbits
      | - Configure the size of the transmit buffer
      | - Configure the size of the reception buffer
      | - Enable/disable the status output port
      mask init:
      | uartChannelInfoStr = sfcn_uart_init_mcb(3, channel, baudrate, databits, parity, stopbits, txbufsize, rxbufsize, useStatusOut);
      settings: CopyFcn=sfcn_uart_init_chk();  MoveFcn=drawLogos
      mask Help: web('sfcn_uart_init.html')
      mask TypeOptions channel: UART1: Con. UEXT-3 & Con. UEXT-4 (PA9 & PA10) | UART2: SUB D9 (PA2 & PA3)
      mask Callback channel: sfcn_uart_init_chk();
      mask TypeOptions baudrate: 300 | 600 | 1200 | 2400 | 4800 | 9600 | 19200 | 38400 | 57600 | 115200
      mask TypeOptions databits: 8 | 9
      mask TypeOptions parity: none | even | odd
      mask TypeOptions stopbits: 1 | 2
      mask Display: fprintf('UART init\n%s', uartChannelInfoStr);patch([236 242 242],[8 14 2],[1 0 0]);patch([244 244 250],[14 2 8],[0 0 0.35]);
  UART receive : Subsystem  Tag=HANcoder_TARGET_STM32_P405  mask(UART receive){channel=UART1: Con. UEXT-3 & Con. UEXT-4 (PA9 & PA10), useStatusOut=off, tsamp=-1}
      mask prompts: useStatusOut "Use status outport"; tsamp "Sample time"
      mask help:
      | Function
      | ==========
      | Reads a byte from the UART reception buffer.
      |
      | Parameters per channel
      | ======================
      | - Select channel
      | - Select if the status output should be enabled.
      |
      | Outputs
      | =======
      | - The value of the receive byte.
      | - When the status output is 0, the reception buffer was empty.
      mask init:
      | uartChannelInfoStr = sfcn_uart_receive_mcb(3, channel, useStatusOut);
      settings: MoveFcn=drawLogos
      mask Help: web('sfcn_uart_receive.html')
      mask TypeOptions channel: UART1: Con. UEXT-3 & Con. UEXT-4 (PA9 & PA10) | UART2: SUB D9 (PA2 & PA3)
      mask Display: fprintf('UART receive\n%s', uartChannelInfoStr);patch([240 246 246],[8 14 2],[1 0 0]);patch([248 248 254],[14 2 8],[0 0 0.35]);
  UART receive buffer status : Subsystem  Tag=HANcoder_TARGET_STM32_P405  mask(UART receive buffer status){channel=UART1: Con. UEXT-3 & Con. UEXT-4 (PA9 & PA10), tsamp=-1}
      mask prompts: tsamp "Sample time"
      mask help:
      | Function
      | ==========
      | Obtains the number of received bytes that are currently stored in the
      | reception buffer.
      |
      | Parameters per channel
      | ======================
      | - Select channel
      |
      | Outputs
      | ======
      | - The number of bytes currently stored in the reception buffer.
      mask init:
      | uartChannelInfoStr = sfcn_uart_receive_size_mcb(3, channel);
      settings: MoveFcn=drawLogos
      mask Help: web('sfcn_uart_receive_size.html')
      mask TypeOptions channel: UART1: Con. UEXT-3 & Con. UEXT-4 (PA9 & PA10) | UART2: SUB D9 (PA2 & PA3)
      mask Display: fprintf('UART receive buffer status\n%s', uartChannelInfoStr);patch([245 251 251],[8 14 2],[1 0 0]);patch([253 253 259],[14 2 8],[0 0 0.35]);
  UART send : Subsystem  Tag=HANcoder_TARGET_STM32_P405  mask(UART send){channel=UART1: Con. UEXT-3 & Con. UEXT-4 (PA9 & PA10), useStatusOut=off, tsamp=-1}
      mask prompts: useStatusOut "Use status outport"; tsamp "Sample time"
      mask help:
      | Function
      | ==========
      | Transmits a byte on the UART communication interface.
      |
      | Parameters per channel
      | ======================
      | - Select channel
      | - Select if the status output should be enabled.
      |
      | Inputs
      | ======
      | - The byte to send
      |
      | Outputs
      | =======
      | - When the status output is 0, the byte could not be transmitted. Probably
      |   because the transmit buffer was configured too small.
      mask init:
      | uartChannelInfoStr = sfcn_uart_send_mcb(3, channel, useStatusOut);
      settings: MoveFcn=drawLogos
      mask Help: web('sfcn_uart_send.html')
      mask TypeOptions channel: UART1: Con. UEXT-3 & Con. UEXT-4 (PA9 & PA10) | UART2: SUB D9 (PA2 & PA3)
      mask Display: fprintf('UART send\n%s', uartChannelInfoStr);patch([245 251 251],[8 14 2],[1 0 0]);patch([253 253 259],[14 2 8],[0 0 0.35]);
